simulink model "SOCPIControlBenchmarkRealDTOptimRand"  (R2019b)
settings: Solver=VariableStepAuto  StartTime=0.0  StopTime=tsim  FixedStep=0.01  RelTol=1e-3
values from neighbouring files (symbols this model uses):
  kio = 0.05    [benchmarkPIDStartRealOptimRand.m]
  kpo = 0.06    [benchmarkPIDStartRealOptimRand.m]
  maxKi = 0.1    [benchmarkPIDStartRealOptimRand.m]
  maxKp = 0.1    [benchmarkPIDStartRealOptimRand.m]
  minKi = 0.001    [benchmarkPIDStartRealOptimRand.m]
  minKp = 0.01    [benchmarkPIDStartRealOptimRand.m]
  optimPeriod = 300    [benchmarkPIDStartRealOptimRand.m]
  OVLim = 2    [benchmarkPIDStartRealOptimRand.m]
  refAmplitude = 50    [benchmarkPIDStartRealOptimRand.m]
  refSignalPeriod = 300    [benchmarkPIDStartRealOptimRand.m]
  resetThreshold = 0.1    [benchmarkPIDStartRealOptimRand.m]
  TSLim = 70    [benchmarkPIDStartRealOptimRand.m]
undefined symbols (not defined in the file or in its folder): conductance, FORandGCNM, resistance
libraries: fl_lib x28, nesl_utility x16, ee_lib x10, commchan3 x2, simulink x2, dspmathops x1
(part 1 of 2)
settings Model: SimulationMode=accelerator  Creator=jairo  LastModifiedBy=jairo
settings DataIOCC: ReturnWorkspaceOutputs=off

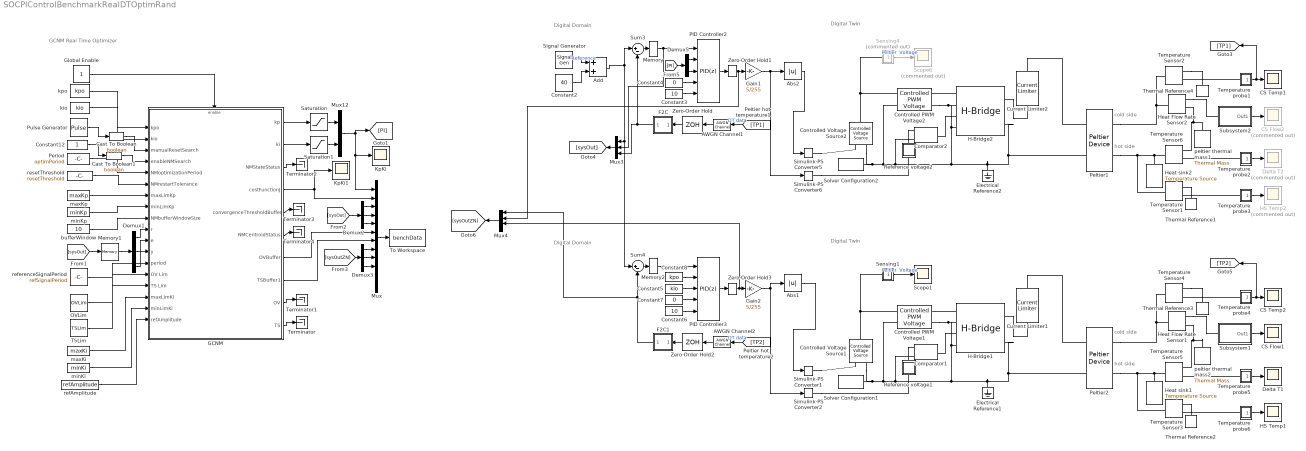
== system SOCPIControlBenchmarkRealDTOptimRand ==
  note: Digital Domain
  note: GCNM Real Time Optimizer
  note: hot side
  note: cold side
  note: Digital Twin
  note: Digital Twin
  note: hot side
  note: Digital Domain
  note: cold side
  AWGN Channel1 : commchan3/AWGN Channel  InputProcessing=Columns as channels (frame based)  seed=20  noiseMode=Variance from mask  EbNodB=10  EsNodB=10  SNRdB=10  bitsPerSym=1  Ps=1  Tsym=1  variance=0.01
      settings: SourceProductName=Communications Toolbox
  AWGN Channel2 : commchan3/AWGN Channel  InputProcessing=Columns as channels (frame based)  seed=20  noiseMode=Variance from mask  EbNodB=10  EsNodB=10  SNRdB=10  bitsPerSym=1  Ps=1  Tsym=1  variance=0.01
      settings: SourceProductName=Communications Toolbox
  Abs1 : Abs
  Abs2 : Abs
  Add : Sum
  CS Flow1 : Scope
  CS Flow2 : Scope  Commented=on
  CS Temp1 : Scope
  CS Temp2 : Scope
  Cast To Boolean : DataTypeConversion  OutDataTypeStr=boolean
  Cast To Boolean1 : DataTypeConversion  OutDataTypeStr=boolean
  Comparator1 : ee_lib/Integrated Circuits/Comparator  V_OS=5 mV  V_OL=0 V  V_OH=5 V  C_IN=0 pF  R_OUT=50 Ohm  Delay=0 s
      settings: SourceProductName=Simscape Electrical  SourceProductBaseCode=PS  InternalSimscapePortConfiguration="{\"Bottom\":[],\"Left\":[{\"id\":\"p\",\"label\":\"+\",\"type\":\"foundation.electrical.electrical\"},{\"id\":\"n\",\"label\":\"-\",\"type\":\"foundation.electrical.electrical\"}],\"Right\":[{\"id\":\"J\",\"label\":\"\",\"type\":\"foundation.electrical.electrical\"}],\"Top\":[]}"
  Comparator2 : ee_lib/Integrated Circuits/Comparator  V_OS=5 mV  V_OL=0 V  V_OH=5 V  C_IN=0 pF  R_OUT=50 Ohm  Delay=0 s
      settings: SourceProductName=Simscape Electrical  SourceProductBaseCode=PS  InternalSimscapePortConfiguration="{\"Bottom\":[],\"Left\":[{\"id\":\"p\",\"label\":\"+\",\"type\":\"foundation.electrical.electrical\"},{\"id\":\"n\",\"label\":\"-\",\"type\":\"foundation.electrical.electrical\"}],\"Right\":[{\"id\":\"J\",\"label\":\"\",\"type\":\"foundation.electrical.electrical\"}],\"Top\":[]}"
  Constant12 : Constant  OutDataTypeStr=boolean
  Constant2 : Constant  Value=40
  Constant3 : Constant  Value=10
  Constant4 : Constant  Value=0
  Constant5 : Constant  Value=kio
  Constant6 : Constant  Value=10
  Constant7 : Constant  Value=0
  Constant8 : Constant  Value=kpo
  Controlled PWM Voltage1 : ee_lib/Integrated Circuits/Controlled PWM Voltage  F=4000 Hz  TD=0 s  pulse_width_offset=0 s  pulse_min=0 s  Vmin=0 V  Vmax=5 V  Vm=5 V  pwm_or_av=2  event_type=1  sample_time=5e-6 s  u_min=0  u_max=1
      settings: SourceProductName=Simscape Electrical
  Controlled PWM Voltage2 : ee_lib/Integrated Circuits/Controlled PWM Voltage  F=4000 Hz  TD=0 s  pulse_width_offset=0 s  pulse_min=0 s  Vmin=0 V  Vmax=5 V  Vm=5 V  pwm_or_av=2  event_type=1  sample_time=5e-6 s  u_min=0  u_max=1
      settings: SourceProductName=Simscape Electrical
  Controlled Voltage Source1 : fl_lib/Electrical/Electrical Sources/Controlled Voltage Source
  Controlled Voltage Source2 : fl_lib/Electrical/Electrical Sources/Controlled Voltage Source
  Current Limiter1 : ee_lib/Semiconductors & Converters/Current Limiter  iLim=5 A  vLim=0.1 V  gLim=1e-3 1/Ohm  thermal_mass=100 J/K  initial_temperature=298.15 K
      settings: SourceProductName=Simscape Electrical  SourceProductBaseCode=PS  InternalSimscapePortConfiguration="{\"Bottom\":[],\"Left\":[{\"id\":\"p\",\"label\":\"+\",\"type\":\"foundation.electrical.electrical\"}],\"Right\":[{\"id\":\"n\",\"label\":\"-\",\"type\":\"foundation.electrical.electrical\"}],\"Top\":[]}"
  Current Limiter2 : ee_lib/Semiconductors & Converters/Current Limiter  iLim=5 A  vLim=0.1 V  gLim=1e-3 1/Ohm  thermal_mass=100 J/K  initial_temperature=298.15 K
      settings: SourceProductName=Simscape Electrical  SourceProductBaseCode=PS  InternalSimscapePortConfiguration="{\"Bottom\":[],\"Left\":[{\"id\":\"p\",\"label\":\"+\",\"type\":\"foundation.electrical.electrical\"}],\"Right\":[{\"id\":\"n\",\"label\":\"-\",\"type\":\"foundation.electrical.electrical\"}],\"Top\":[]}"
  Delta T1 : Scope
  Delta T2 : Scope  Commented=on
  Demux1 : Demux  Outputs=3
  Demux2 : Demux  Outputs=3
  Demux3 : Demux  Outputs=3
  Demux5 : Demux  Outputs=2
  Electrical Reference1 : fl_lib/Electrical/Electrical Elements/Electrical Reference
  Electrical Reference2 : fl_lib/Electrical/Electrical Elements/Electrical Reference
  F2C : Subsystem
  F2C1 : Subsystem
  GCNM : Subsystem
  Gain1 : Gain  Gain=5/255
  Gain2 : Gain  Gain=5/255
  Global Enable : Constant
  H-Bridge1 : ee_lib/Semiconductors & Converters/Converters/H-Bridge  supply_ports=ee.enum.supply_ports.hidesupply  Venable=2.5 V  Vmax=5 V  Vreverse=0.1 V  Vbrake=2.5 V  Vm=12 V  pwm_or_av=ee.enum.pwm_or_av.averaged  regenerative_braking_mode=ee.enum.converters.regenerative_braking_mode.always_enabled  discontinuous=ee.enum.current_profile.continuous  freewheeling_mode=ee.enum.converters.freewheeling_mode.one_switch_one_diode  Ron=0.1 Ohm  Don=0.1 Ohm  Goff=1e-6 S  Rload=3.38+0.1 Ohm  Lload=1e-5 H  F=4 kHz  thermal_mass=100 J/K  initial_temperature=298.15 K  Ron2=0.1 Ohm  Don2=0.05 Ohm  Tmeas=298.15 K  Tmeas2=398.15 K
      settings: SourceProductName=Simscape Electrical
  H-Bridge2 : ee_lib/Semiconductors & Converters/Converters/H-Bridge  supply_ports=ee.enum.supply_ports.hidesupply  Venable=2.5 V  Vmax=5 V  Vreverse=0.1 V  Vbrake=2.5 V  Vm=12 V  pwm_or_av=ee.enum.pwm_or_av.averaged  regenerative_braking_mode=ee.enum.converters.regenerative_braking_mode.always_enabled  discontinuous=ee.enum.current_profile.continuous  freewheeling_mode=ee.enum.converters.freewheeling_mode.one_switch_one_diode  Ron=0.1 Ohm  Don=0.1 Ohm  Goff=1e-6 S  Rload=3.38+0.1 Ohm  Lload=1e-5 H  F=4 kHz  thermal_mass=100 J/K  initial_temperature=298.15 K  Ron2=0.1 Ohm  Don2=0.05 Ohm  Tmeas=298.15 K  Tmeas2=398.15 K
      settings: SourceProductName=Simscape Electrical
  HS Temp1 : Scope
  HS Temp2 : Scope  Commented=on
  Heat Flow Rate Sensor1 : fl_lib/Thermal/Thermal Sensors/Heat Flow Rate Sensor
      settings: SourceProductName=Simscape  SourceProductBaseCode=SS
  Heat Flow Rate Sensor2 : fl_lib/Thermal/Thermal Sensors/Heat Flow Rate Sensor
      settings: SourceProductName=Simscape  SourceProductBaseCode=SS
  Heat sink1 : fl_lib/Thermal/Thermal Sources/Temperature Source  temperature=296 K
      settings: SourceProductName=Simscape
  Heat sink2 : fl_lib/Thermal/Thermal Sources/Temperature Source  temperature=296 K
      settings: SourceProductName=Simscape
  KpKi : Scope
  KpKi1 : Scope
  Memory : Memory
  Memory1 : Memory
  Memory2 : Memory
  Mux : Mux  Inputs=12
  Mux12 : Mux  Inputs=2
  Mux3 : Mux  Inputs=3
  Mux4 : Mux
  OVLim : Constant  Value=OVLim
  PID Controller2 : simulink/Continuous/PID Controller  Controller=PID  Form=Parallel  TimeDomain=Discrete-time  SampleTime=0.01  IntegratorMethod=Forward Euler  FilterMethod=Forward Euler  ControllerParametersSource=external  P=38.57  I=1.46877  D=6.66875  UseFilter=on  N=100  TunerSelectOption=Transfer Function Based (PID Tuner App)  InitialConditionSource=internal  InitialConditionForIntegrator=0  InitialConditionForFilter=0  DifferentiatorICPrevScaledInput=0  ExternalReset=none  TrackingMode=off  Kt=1  LimitOutput=on  UpperSaturationLimit=255  LowerSaturationLimit=-255  LinearizeAsGain=on  AntiWindupMode=back-calculation  Kb=1  POutMin=[]  POutMax=[]  IOutMin=[]  IOutMax=[]  DOutMin=[]  DOutMax=[]  NOutMin=[]  NOutMax=[]  SumOutMin=[]  SumOutMax=[]  SaturationOutMin=[]  SaturationOutMax=[]  PParamMin=[]  PParamMax=[]  IParamMin=[]  IParamMax=[]  DParamMin=[]  DParamMax=[]  NParamMin=[]  NParamMax=[]  KbParamMin=[]  KbParamMax=[]  KtParamMin=[]  KtParamMax=[]  KbOutMin=[]  KbOutMax=[]  KtOutMin=[]  KtOutMax=[]  IntegratorOutMin=[]  IntegratorOutMax=[]  FilterOutMin=[]  FilterOutMax=[]  SumI1OutMin=[]  SumI1OutMax=[]  SumI2OutMin=[]  SumI2OutMax=[]  SumI3OutMin=[]  SumI3OutMax=[]  SumI4OutMin=[]  SumI4OutMax=[]  SumDOutMin=[]  SumDOutMax=[]  DifferentiatorOutMin=[]  DifferentiatorOutMax=[]  FilterDiffOutCoefMin=[]  FilterDiffOutCoefMax=[]  ReciprocalOutMin=[]  ReciprocalOutMax=[]  SumDenOutMin=[]  SumDenOutMax=[]  SumNumOutMin=[]  SumNumOutMax=[]  DivideOutMin=[]  DivideOutMax=[]  IntegratorContinuousStateAttributes=''  IntegratorStateMustResolveToSignalObject=off  IntegratorRTWStateStorageClass=Auto  FilterContinuousStateAttributes=''  FilterStateMustResolveToSignalObject=off  FilterRTWStateStorageClass=Auto  ParallelPVariant=ExternalParameters  IdealPVariant=Disabled  IVariant=ExternalParameters  DVariant=ExternalParameters  IntegratorVariant=Discrete  SatVariant=Enabled  AWVariant=BackCalculation  PCopyVariant=Disabled  TRVariant=Disabled  FdbkBlocksVariant=Forward  IdealPFdbkVariant=Disabled  SatFdbkVariant=Disabled  DerivativeFilterVariant=ForwardEulerFilter  NVariant=ExternalParameters  NCopyVariant=Disabled  FilterICVariant=InternalICsFilter  IntegratorICVariant=InternalICs  ExternalResetVariant=Disabled  TRSumVariant=Passthrough  SumFdbkVariant=Disabled  SumVariant=Sum_PID
  PID Controller3 : simulink/Continuous/PID Controller  Controller=PID  Form=Parallel  TimeDomain=Discrete-time  SampleTime=0.01  IntegratorMethod=Forward Euler  FilterMethod=Forward Euler  ControllerParametersSource=external  P=38.57  I=1.46877  D=6.66875  UseFilter=on  N=100  TunerSelectOption=Transfer Function Based (PID Tuner App)  InitialConditionSource=internal  InitialConditionForIntegrator=0  InitialConditionForFilter=0  DifferentiatorICPrevScaledInput=0  ExternalReset=none  TrackingMode=off  Kt=1  LimitOutput=on  UpperSaturationLimit=255  LowerSaturationLimit=-255  LinearizeAsGain=on  AntiWindupMode=back-calculation  Kb=1  POutMin=[]  POutMax=[]  IOutMin=[]  IOutMax=[]  DOutMin=[]  DOutMax=[]  NOutMin=[]  NOutMax=[]  SumOutMin=[]  SumOutMax=[]  SaturationOutMin=[]  SaturationOutMax=[]  PParamMin=[]  PParamMax=[]  IParamMin=[]  IParamMax=[]  DParamMin=[]  DParamMax=[]  NParamMin=[]  NParamMax=[]  KbParamMin=[]  KbParamMax=[]  KtParamMin=[]  KtParamMax=[]  KbOutMin=[]  KbOutMax=[]  KtOutMin=[]  KtOutMax=[]  IntegratorOutMin=[]  IntegratorOutMax=[]  FilterOutMin=[]  FilterOutMax=[]  SumI1OutMin=[]  SumI1OutMax=[]  SumI2OutMin=[]  SumI2OutMax=[]  SumI3OutMin=[]  SumI3OutMax=[]  SumI4OutMin=[]  SumI4OutMax=[]  SumDOutMin=[]  SumDOutMax=[]  DifferentiatorOutMin=[]  DifferentiatorOutMax=[]  FilterDiffOutCoefMin=[]  FilterDiffOutCoefMax=[]  ReciprocalOutMin=[]  ReciprocalOutMax=[]  SumDenOutMin=[]  SumDenOutMax=[]  SumNumOutMin=[]  SumNumOutMax=[]  DivideOutMin=[]  DivideOutMax=[]  IntegratorContinuousStateAttributes=''  IntegratorStateMustResolveToSignalObject=off  IntegratorRTWStateStorageClass=Auto  FilterContinuousStateAttributes=''  FilterStateMustResolveToSignalObject=off  FilterRTWStateStorageClass=Auto  ParallelPVariant=ExternalParameters  IdealPVariant=Disabled  IVariant=ExternalParameters  DVariant=ExternalParameters  IntegratorVariant=Discrete  SatVariant=Enabled  AWVariant=BackCalculation  PCopyVariant=Disabled  TRVariant=Disabled  FdbkBlocksVariant=Forward  IdealPFdbkVariant=Disabled  SatFdbkVariant=Disabled  DerivativeFilterVariant=ForwardEulerFilter  NVariant=ExternalParameters  NCopyVariant=Disabled  FilterICVariant=InternalICsFilter  IntegratorICVariant=InternalICs  ExternalResetVariant=Disabled  TRSumVariant=Passthrough  SumFdbkVariant=Disabled  SumVariant=Sum_PID
  Peltier1 : ee_lib/Sensors & Transducers/Peltier Device  alpha=seebeck V/K  R=resistance Ohm  K=conductance W/K
      settings: SourceProductName=Simscape Electrical  SourceProductBaseCode=PS  InternalSimscapePortConfiguration="{\"Bottom\":[],\"Left\":[{\"id\":\"p\",\"label\":\"+\",\"type\":\"foundation.electrical.electrical\"},{\"id\":\"n\",\"label\":\"-\",\"type\":\"foundation.electrical.electrical\"}],\"Right\":[{\"id\":\"A\",\"label\":\"A\",\"type\":\"foundation.thermal.thermal\"},{\"id\":\"B\",\"label\":\"B\",\"type\":\"foundation.thermal.thermal\"}],\"Top\":[]}"
  Peltier2 : ee_lib/Sensors & Transducers/Peltier Device  alpha=seebeck V/K  R=resistance Ohm  K=conductance W/K
      settings: SourceProductName=Simscape Electrical  SourceProductBaseCode=PS  InternalSimscapePortConfiguration="{\"Bottom\":[],\"Left\":[{\"id\":\"p\",\"label\":\"+\",\"type\":\"foundation.electrical.electrical\"},{\"id\":\"n\",\"label\":\"-\",\"type\":\"foundation.electrical.electrical\"}],\"Right\":[{\"id\":\"A\",\"label\":\"A\",\"type\":\"foundation.thermal.thermal\"},{\"id\":\"B\",\"label\":\"B\",\"type\":\"foundation.thermal.thermal\"}],\"Top\":[]}"
  Period : Constant  Value=optimPeriod  OutDataTypeStr=double
  Pulse Generator : DiscretePulseGenerator  PulseType=Time based  Period=20  PulseWidth=0.1
  Reference voltage1 : Subsystem
      mask Display: disp('Vr')
  Reference voltage2 : Subsystem
      mask Display: disp('Vr')
  Saturation : Saturate  UpperLimit=200  LowerLimit=0
  Saturation1 : Saturate  UpperLimit=200  LowerLimit=0
  Scope1 : Scope
  Scope6 : Scope  Commented=on
  Sensing1 : Subsystem
      mask Display: disp('V')
  Sensing4 : Subsystem  Commented=on
      mask Display: disp('V')
  Signal Generator : SignalGenerator  WaveForm=square  Amplitude=10  Frequency=1/refSignalPeriod
  Simulink-PS Converter{1..2,5..6} (4 alike) : nesl_utility/Simulink-PS Converter  PhysicalDomain=network_engine_domain  SubClassName=ps_input  LeftPortType=input  RightPortType=output  PseudoPeriodic=off  Frequencies=[]  NoiseDistribution=none  NoiseParameters=[]  Unit=1  AffineConversion=off  FilteringAndDerivatives=provide  SimscapeFilterOrder=1  InputFilterTimeConstant=0.001  UdotUserProvided=0
  Solver Configuration1 : nesl_utility/Solver Configuration  PhysicalDomain=network_engine_domain  SubClassName=solver  LeftPortType=input  RightPortType=generic  Tones=[]  Harmonics=[]  SimulateNoise=off  Profile=off  UseLocalSampling=off  EnableSwitchedLinearOptims=on  FrequencyDomain=off  UseCCode=off  RelTol=0.001  AbsTol=1e-06  MinStep=1e-09  ToWorkspace=off  RevertToSquareIcSolve=off  NumHomotopyIterations=100  PhasorMode=off  PhasorModeNumHarmonics=1  DoDC=off  ResidualTolerance=1e-09  UseLocalSolver=off  LocalSolverChoice=NE_BACKWARD_EULER_ADVANCER  LocalSolverSampleTime=0.001  DoFixedCost=off  MaxNonlinIter=3  MaxModeIter=2  LinearAlgebra=auto  EquationFormulation=NE_TIME_EF  DelaysMemoryBudget=1024  AutomaticFiltering=on  FilteringTimeConstant=0.01  PartitionStorageMethod=AS_NEEDED  PartitionMemoryBudget=1024  PartitionMethod=FAST
  Solver Configuration2 : nesl_utility/Solver Configuration  PhysicalDomain=network_engine_domain  SubClassName=solver  LeftPortType=input  RightPortType=generic  Tones=[]  Harmonics=[]  SimulateNoise=off  Profile=off  UseLocalSampling=off  EnableSwitchedLinearOptims=on  FrequencyDomain=off  UseCCode=off  RelTol=0.001  AbsTol=1e-06  MinStep=1e-09  ToWorkspace=off  RevertToSquareIcSolve=off  NumHomotopyIterations=100  PhasorMode=off  PhasorModeNumHarmonics=1  DoDC=off  ResidualTolerance=1e-09  UseLocalSolver=off  LocalSolverChoice=NE_BACKWARD_EULER_ADVANCER  LocalSolverSampleTime=0.001  DoFixedCost=off  MaxNonlinIter=3  MaxModeIter=2  LinearAlgebra=auto  EquationFormulation=NE_TIME_EF  DelaysMemoryBudget=1024  AutomaticFiltering=on  FilteringTimeConstant=0.01  PartitionStorageMethod=AS_NEEDED  PartitionMemoryBudget=1024  PartitionMethod=FAST
  Subsystem1 : Subsystem
      mask Display: disp('Heat flow')
  Subsystem2 : Subsystem
      mask Display: disp('Heat flow')
  Sum3 : Sum  Inputs=|+-
  Sum4 : Sum  Inputs=|+-
  TSLim : Constant  Value=TSLim
  Temperature Sensor{1..6} (6 alike) : fl_lib/Thermal/Thermal Sensors/Temperature Sensor
  Temperature probe1 : Subsystem
      mask Display: disp('T')
  Temperature probe2 : Subsystem
      mask Display: disp('T')
  Temperature probe3 : Subsystem
      mask Display: disp('T')
  Temperature probe4 : Subsystem
      mask Display: disp('T')
  Temperature probe5 : Subsystem
      mask Display: disp('T')
  Temperature probe6 : Subsystem
      mask Display: disp('T')
  Terminator{,1..4} (5 alike) : Terminator
  Thermal Reference{1..4} (4 alike) : fl_lib/Thermal/Thermal Elements/Thermal Reference
  To Workspace : ToWorkspace  VariableName=benchData  SaveFormat=Timeseries  SampleTime=-1
  Zero-Order Hold : ZeroOrderHold  SampleTime=-1
  Zero-Order Hold1 : ZeroOrderHold
  Zero-Order Hold2 : ZeroOrderHold  SampleTime=-1
  Zero-Order Hold3 : ZeroOrderHold
  bufferWindow : Constant  Value=10  OutDataTypeStr=uint16
  kio : Constant  Value=kio  OutDataTypeStr=double
  kpo : Constant  Value=kpo  OutDataTypeStr=double
  maxKi : Constant  Value=maxKi  VectorParams1D=off  OutDataTypeStr=double
  maxKp : Constant  Value=maxKp  OutDataTypeStr=double
  minKi : Constant  Value=minKi  OutDataTypeStr=double
  minKp : Constant  Value=minKp  OutDataTypeStr=double
  peltier thermal mass1 : fl_lib/Thermal/Thermal Elements/Thermal Mass  mass=1 kg  sp_heat=Cp J/kg/K  T_specify=on  T_priority=High  T=296 K  T_nominal_specify=off  T_nominal_unit=K  T_nominal_value=1  Q_specify=off  Q_priority=Low  Q=0 W  Q_nominal_specify=off  Q_nominal_unit=W  Q_nominal_value=1
  peltier thermal mass2 : fl_lib/Thermal/Thermal Elements/Thermal Mass  mass=1 kg  sp_heat=Cp J/kg/K  T_specify=on  T_priority=High  T=296 K  T_nominal_specify=off  T_nominal_unit=K  T_nominal_value=1  Q_specify=off  Q_priority=Low  Q=0 W  Q_nominal_specify=off  Q_nominal_unit=W  Q_nominal_value=1
  refAmplitude : Constant  Value=refAmplitude  OutDataTypeStr=double
  referenceSignalPeriod : Constant  Value=refSignalPeriod
  resetThreshold : Constant  Value=resetThreshold
  wires:
  resetThreshold/1 -> GCNM/6(NMrestartTolerance)
  Mux12/1 -> [PI], Mux/1, KpKi/1
  maxKp/1 -> GCNM/7(maxLimKp)
  bufferWindow/1 -> GCNM/9(NMbufferWindowSize)
  Cast To Boolean1/1 -> GCNM/4(enableNMSearch)
  kio/1 -> GCNM/2(kio)
  Pulse Generator/1 -> Cast To Boolean/1
  Cast To Boolean/1 -> GCNM/3(manualResetSearch)
  Constant12/1 -> Cast To Boolean1/1
  minKp/1 -> GCNM/8(minLimKp)
  Global Enable/1 -> GCNM/Enable
  kpo/1 -> GCNM/1(kpo)
  Period/1 -> GCNM/5(NMoptimizationPeriod)
  GCNM/4(costFunctionJ) -> Mux/2, KpKi1/1
  referenceSignalPeriod/1 -> GCNM/13("  period")
  OVLim/1 -> GCNM/14("  OV Lim")
  TSLim/1 -> GCNM/15(TS Lim)
  GCNM/1("  kp") -> Saturation/1
  GCNM/2("  ki") -> Saturation1/1
  Mux/1 -> To Workspace/1
  maxKi/1 -> GCNM/16(maxLimKi)
  minKi/1 -> GCNM/17(minLimKi)
  [sysOut] -> Memory1/1
  Demux1/1 -> GCNM/10("  r")
  Demux1/2 -> GCNM/11("  e")
  Demux1/3 -> GCNM/12("  y")
  [sysOut] -> Demux2/1
  Demux2/1 -> Mux/3
  Demux2/2 -> Mux/4
  Demux2/3 -> Mux/5
  [sysOutZN] -> Demux3/1
  Demux3/1 -> Mux/8
  Demux3/2 -> Mux/9
  Demux3/3 -> Mux/10
  GCNM/10(TS) -> Terminator/1
  GCNM/9(OV) -> Terminator1/1
  GCNM/8(TSBuffer1) -> Mux/7
  GCNM/7(OVBuffer) -> Mux/6
  GCNM/3(NMStateStatus) -> Terminator2/1
  GCNM/5(convergenceThresholdBuffer) -> Terminator3/1
  GCNM/6(NMCentroidStatus) -> Terminator4/1
  Signal Generator/1 -> Add/1  "Reference"
  Constant2/1 -> Add/2
  refAmplitude/1 -> GCNM/18(refAmplitude)
  Sensing4/1(Out1) -> Scope6/1  "Peltier  Voltage"
  Zero-Order Hold1/1 -> Mux4/2, Gain1/1
  Temperature probe1/1(K) -> [TP1], CS Temp1/1
  [TP1] -> AWGN Channel1/1  "DT data"
  PID Controller2/1 -> Zero-Order Hold1/1
  Temperature probe2/1(K) -> Delta T2/1
  Subsystem2/1(Out1) -> CS Flow2/1
  Gain1/1 -> Abs2/1, Simulink-PS Converter6/1
  Abs2/1 -> Simulink-PS Converter5/1
  Temperature probe3/1(K) -> HS Temp2/1
  AWGN Channel1/1 -> Zero-Order Hold/1
  Mux3/1 -> [sysOut]
  Constant4/1 -> PID Controller2/4
  Constant3/1 -> PID Controller2/5
  Zero-Order Hold/1 -> F2C/1(In1)
  Sum3/1 -> Memory/1
  Memory/1 -> Mux3/2, PID Controller2/1
  [PI] -> Demux5/1
  Demux5/1 -> PID Controller2/2
  Demux5/2 -> PID Controller2/3
  Memory1/1 -> Demux1/1
  F2C/1(Out1) -> Mux3/3, Sum3/2
  Temperature probe5/1(K) -> Delta T1/1
  PID Controller3/1 -> Zero-Order Hold3/1
  Zero-Order Hold3/1 -> Mux4/3, Gain2/1
  Temperature probe4/1(K) -> [TP2], CS Temp2/1
  Sensing1/1(Out1) -> Scope1/1  "Peltier  Voltage"
  Sum4/1 -> Memory2/1
  Abs1/1 -> Simulink-PS Converter1/1
  AWGN Channel2/1 -> Zero-Order Hold2/1
  Add/1 -> Sum4/1, Mux3/1, Sum3/1
  Gain2/1 -> Abs1/1, Simulink-PS Converter2/1
  Zero-Order Hold2/1 -> F2C1/1(In1)
  Subsystem1/1(Out1) -> CS Flow1/1
  [TP2] -> AWGN Channel2/1  "DT data"
  F2C1/1(Out1) -> Mux4/1, Sum4/2
  Constant7/1 -> PID Controller3/4
  Memory2/1 -> PID Controller3/1
  Temperature probe6/1(K) -> HS Temp1/1
  Constant6/1 -> PID Controller3/5
  Mux4/1 -> [sysOutZN]
  Constant8/1 -> PID Controller3/2
  Constant5/1 -> PID Controller3/3
  Saturation/1 -> Mux12/1
  Saturation1/1 -> Mux12/2
  connections:
  Controlled PWM Voltage2/LConn1 -- Controlled Voltage Source2/LConn1 -- Sensing4/LConn1
  Peltier1/RConn1 -- Heat Flow Rate Sensor2/LConn1 -- Temperature Sensor2/LConn1
  Controlled PWM Voltage2/RConn2 -- Peltier1/LConn2 -- H-Bridge2/RConn2 -- Electrical Reference2/LConn1 -- Comparator2/LConn2 -- Controlled Voltage Source2/RConn2 -- Solver Configuration2/RConn1 -- Controlled PWM Voltage2/LConn2 -- H-Bridge2/LConn4 -- H-Bridge2/LConn2
  peltier thermal mass1/LConn1 -- Temperature Sensor6/RConn1 -- Heat Flow Rate Sensor2/RConn2
  Heat sink2/LConn1 -- Temperature Sensor6/LConn1 -- Peltier1/RConn2 -- Temperature Sensor1/LConn1
  Peltier1/LConn1 -- Current Limiter2/RConn1
  Simulink-PS Converter6/RConn1 -- Reference voltage2/RConn1
  Temperature Sensor2/RConn1 -- Thermal Reference4/LConn1
  Temperature Sensor1/RConn1 -- Thermal Reference1/LConn1
  Heat Flow Rate Sensor2/RConn1 -- Subsystem2/LConn1
  Comparator2/RConn1 -- H-Bridge2/LConn3
  Reference voltage2/LConn1 -- Comparator2/LConn1
  Temperature probe1/LConn1 -- Temperature Sensor2/RConn2
  Temperature probe3/LConn1 -- Temperature Sensor1/RConn2
  Temperature probe2/LConn1 -- Temperature Sensor6/RConn2
  H-Bridge2/RConn1 -- Current Limiter2/LConn1
  Simulink-PS Converter5/RConn1 -- Controlled Voltage Source2/RConn1
  H-Bridge2/LConn1 -- Controlled PWM Voltage2/RConn1
  Controlled PWM Voltage1/RConn2 -- H-Bridge1/LConn2 -- H-Bridge1/LConn4 -- Peltier2/LConn2 -- H-Bridge1/RConn2 -- Electrical Reference1/LConn1 -- Comparator1/LConn2 -- Controlled Voltage Source1/RConn2 -- Solver Configuration1/RConn1 -- Controlled PWM Voltage1/LConn2
  Heat sink1/LConn1 -- Temperature Sensor5/LConn1 -- Peltier2/RConn2 -- Temperature Sensor3/LConn1
  Peltier2/RConn1 -- Heat Flow Rate Sensor1/LConn1 -- Temperature Sensor4/LConn1
  peltier thermal mass2/LConn1 -- Temperature Sensor5/RConn1 -- Heat Flow Rate Sensor1/RConn2
  Controlled PWM Voltage1/LConn1 -- Controlled Voltage Source1/LConn1 -- Sensing1/LConn1
  Peltier2/LConn1 -- Current Limiter1/RConn1
  Temperature probe4/LConn1 -- Temperature Sensor4/RConn2
  Heat Flow Rate Sensor1/RConn1 -- Subsystem1/LConn1
  Temperature Sensor3/RConn1 -- Thermal Reference2/LConn1
  Temperature Sensor4/RConn1 -- Thermal Reference3/LConn1
  Reference voltage1/LConn1 -- Comparator1/LConn1
  Simulink-PS Converter2/RConn1 -- Reference voltage1/RConn1
  H-Bridge1/LConn1 -- Controlled PWM Voltage1/RConn1
  Temperature probe5/LConn1 -- Temperature Sensor5/RConn2
  Comparator1/RConn1 -- H-Bridge1/LConn3
  H-Bridge1/RConn1 -- Current Limiter1/LConn1
  Temperature probe6/LConn1 -- Temperature Sensor3/RConn2
  Simulink-PS Converter1/RConn1 -- Controlled Voltage Source1/RConn1

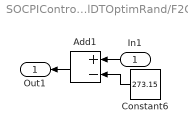
== system SOCPIControlBenchmarkRealDTOptimRand/F2C ==
  In1 : Inport
  Add1 : Sum  Inputs=+-
  Constant6 : Constant  Value=273.15
  Out1 : Outport
  wires:
  Add1/1 -> Out1/1
  Constant6/1 -> Add1/2
  In1/1 -> Add1/1

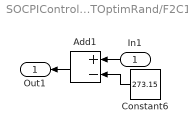
== system SOCPIControlBenchmarkRealDTOptimRand/F2C1 ==
  In1 : Inport
  Add1 : Sum  Inputs=+-
  Constant6 : Constant  Value=273.15
  Out1 : Outport
  wires:
  Add1/1 -> Out1/1
  Constant6/1 -> Add1/2
  In1/1 -> Add1/1

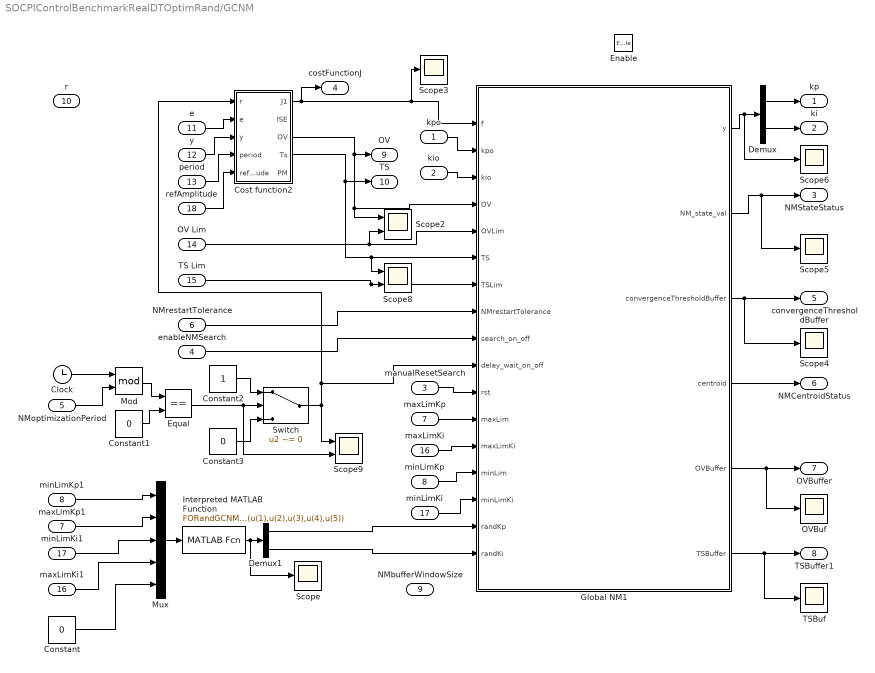
== system SOCPIControlBenchmarkRealDTOptimRand/GCNM ==
  kpo : Inport  OutDataTypeStr=double
  kio : Inport  Port=2  OutDataTypeStr=double
  manualResetSearch : Inport  Port=3  OutDataTypeStr=boolean
  enableNMSearch : Inport  Port=4  OutDataTypeStr=boolean
  NMoptimizationPeriod : Inport  Port=5  OutDataTypeStr=double
  NMrestartTolerance : Inport  Port=6
  maxLimKp : Inport  Port=7  OutDataTypeStr=double
  minLimKp : Inport  Port=8  OutDataTypeStr=double
  NMbufferWindowSize : Inport  Port=9  OutDataTypeStr=uint16
  "  r" : Inport  Port=10  OutDataTypeStr=double
  "  e" : Inport  Port=11  OutDataTypeStr=double
  "  y" : Inport  Port=12  OutDataTypeStr=double
  "  period" : Inport  Port=13  OutDataTypeStr=double
  "  OV Lim" : Inport  Port=14  OutDataTypeStr=double
  TS Lim : Inport  Port=15  OutDataTypeStr=double
  maxLimKi : Inport  Port=16  OutDataTypeStr=double
  minLimKi : Inport  Port=17  OutDataTypeStr=double
  refAmplitude : Inport  Port=18  OutDataTypeStr=double
  Enable : EnablePort
  Clock : Clock
  Constant : Constant  Value=0
  Constant1 : Constant  Value=0
  Constant2 : Constant
  Constant3 : Constant  Value=0
  Cost function2 : Subsystem
  Demux : Demux  Outputs=2
  Demux1 : Demux  Outputs=2
  Equal : RelationalOperator  Operator===  RndMeth=Simplest
  Global NM1 : MATLAB Function  TreatAsAtomicUnit=on
  Interpreted MATLAB Function : MATLABFcn  MATLABFcn=FORandGCNM(u(1),u(2),u(3),u(4),u(5))  OutputDimensions=2
  Mod : Math  Operator=mod  SignedPower=off  SaturateOnIntegerOverflow=on
  Mux : Mux  Inputs=5
  OVBuf : Scope
  Scope{,3..6} (5 alike) : Scope
  Scope2 : Scope  NumInputPorts=2
  Scope8 : Scope  NumInputPorts=2
  Scope9 : Scope  NumInputPorts=2
  Switch : Switch  Criteria=u2 ~= 0
  TSBuf : Scope
  maxLimKi1 : InportShadow  Port=16  OutDataTypeStr=double
  maxLimKp1 : InportShadow  Port=7  OutDataTypeStr=double
  minLimKi1 : InportShadow  Port=17  OutDataTypeStr=double
  minLimKp1 : InportShadow  Port=8  OutDataTypeStr=double
  "  kp" : Outport  OutDataTypeStr=double
  "  ki" : Outport  Port=2  OutDataTypeStr=double
  NMStateStatus : Outport  Port=3  OutDataTypeStr=double
  costFunctionJ : Outport  Port=4  OutDataTypeStr=double
  convergenceThresholdBuffer : Outport  Port=5  OutDataTypeStr=double
  NMCentroidStatus : Outport  Port=6  OutDataTypeStr=double
  OVBuffer : Outport  Port=7  OutDataTypeStr=double
  TSBuffer1 : Outport  Port=8  OutDataTypeStr=double
  OV : Outport  Port=9  OutDataTypeStr=double
  TS : Outport  Port=10  OutDataTypeStr=double
  wires:
  Demux/2 -> "  ki"/1
  Demux/1 -> "  kp"/1
  NMrestartTolerance/1 -> Global NM1/8(NMrestartTolerance)
  manualResetSearch/1 -> Global NM1/11(rst)
  enableNMSearch/1 -> Global NM1/9(search_on_off)
  minLimKp/1 -> Global NM1/14(minLim)
  maxLimKp/1 -> Global NM1/12(maxLim)
  Global NM1/2(NM_state_val) -> Scope5/1, NMStateStatus/1
  Global NM1/3(convergenceThresholdBuffer) -> Scope4/1, convergenceThresholdBuffer/1
  Global NM1/4(centroid) -> NMCentroidStatus/1
  Global NM1/1(y) -> Scope6/1, Demux/1
  kpo/1 -> Global NM1/2(kpo)
  kio/1 -> Global NM1/3(kio)
  Cost function2/3(OV) -> OV/1, Global NM1/4(OV), Scope2/1
  "  y"/1 -> Cost function2/3(y)
  "  e"/1 -> Cost function2/2(e)
  Global NM1/5(OVBuffer) -> OVBuf/1, OVBuffer/1
  "  period"/1 -> Cost function2/4(period)
  "  OV Lim"/1 -> Scope2/2, Global NM1/5(OVLim)
  Cost function2/4(Ts) -> TS/1, Global NM1/6(TS), Scope8/1
  TS Lim/1 -> Global NM1/7(TSLim), Scope8/2
  Global NM1/6(TSBuffer) -> TSBuf/1, TSBuffer1/1
  Cost function2/1(J1) -> Scope3/1, Global NM1/1(f), costFunctionJ/1
  Clock/1 -> Mod/1
  NMoptimizationPeriod/1 -> Mod/2
  Constant1/1 -> Equal/2
  Mod/1 -> Equal/1
  Constant2/1 -> Switch/1
  Constant3/1 -> Switch/3
  Switch/1 -> Scope9/1, Cost function2/1(r), Global NM1/10(delay_wait_on_off)
  Equal/1 -> Scope9/2, Switch/2
  maxLimKi/1 -> Global NM1/13(maxLimKi)
  minLimKi/1 -> Global NM1/15(minLimKi)
  refAmplitude/1 -> Cost function2/5(refAmplitude)
  Mux/1 -> Interpreted MATLAB Function/1
  minLimKp1/1 -> Mux/1
  maxLimKp1/1 -> Mux/2
  Interpreted MATLAB Function/1 -> Scope/1, Demux1/1
  Demux1/1 -> Global NM1/16(randKp)
  Demux1/2 -> Global NM1/17(randKi)
  Constant/1 -> Mux/5
  maxLimKi1/1 -> Mux/4
  minLimKi1/1 -> Mux/3

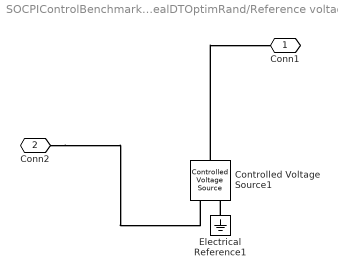
== system SOCPIControlBenchmarkRealDTOptimRand/Reference voltage1 ==
  Controlled Voltage Source1 : fl_lib/Electrical/Electrical Sources/Controlled Voltage Source
  Electrical Reference1 : fl_lib/Electrical/Electrical Elements/Electrical Reference
  Conn1 : PMIOPort  Side=Left
  Conn2 : PMIOPort  Port=2  Side=Right
  connections:
  Electrical Reference1/LConn1 -- Controlled Voltage Source1/RConn2
  Controlled Voltage Source1/LConn1 -- Conn1/RConn1
  Conn2/RConn1 -- Controlled Voltage Source1/RConn1

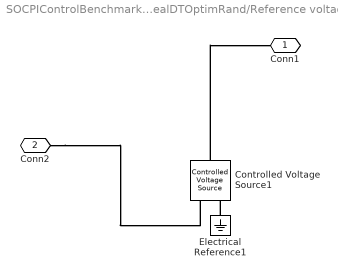
== system SOCPIControlBenchmarkRealDTOptimRand/Reference voltage2 ==
  Controlled Voltage Source1 : fl_lib/Electrical/Electrical Sources/Controlled Voltage Source
  Electrical Reference1 : fl_lib/Electrical/Electrical Elements/Electrical Reference
  Conn1 : PMIOPort  Side=Left
  Conn2 : PMIOPort  Port=2  Side=Right
  connections:
  Electrical Reference1/LConn1 -- Controlled Voltage Source1/RConn2
  Controlled Voltage Source1/LConn1 -- Conn1/RConn1
  Conn2/RConn1 -- Controlled Voltage Source1/RConn1

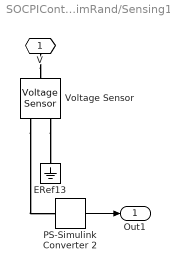
== system SOCPIControlBenchmarkRealDTOptimRand/Sensing1 ==
  ERef13 : fl_lib/Electrical/Electrical Elements/Electrical Reference
  PS-Simulink Converter 2 : nesl_utility/PS-Simulink Converter  PhysicalDomain=network_engine_domain  SubClassName=ps_output  LeftPortType=input  RightPortType=output  PseudoPeriodic=off  Frequencies=[]  Unit=V  AffineConversion=off
  Voltage Sensor : fl_lib/Electrical/Electrical Sensors/Voltage Sensor
  V : PMIOPort  Side=Left
  Out1 : Outport  VectorParamsAs1DForOutWhenUnconnected=off
  wires:
  PS-Simulink Converter 2/1 -> Out1/1
  connections:
  V/RConn1 -- Voltage Sensor/LConn1
  Voltage Sensor/RConn2 -- ERef13/LConn1
  Voltage Sensor/RConn1 -- PS-Simulink Converter 2/LConn1

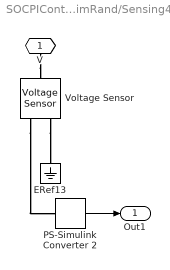
== system SOCPIControlBenchmarkRealDTOptimRand/Sensing4 ==
  ERef13 : fl_lib/Electrical/Electrical Elements/Electrical Reference
  PS-Simulink Converter 2 : nesl_utility/PS-Simulink Converter  PhysicalDomain=network_engine_domain  SubClassName=ps_output  LeftPortType=input  RightPortType=output  PseudoPeriodic=off  Frequencies=[]  Unit=V  AffineConversion=off
  Voltage Sensor : fl_lib/Electrical/Electrical Sensors/Voltage Sensor
  V : PMIOPort  Side=Left
  Out1 : Outport  VectorParamsAs1DForOutWhenUnconnected=off
  wires:
  PS-Simulink Converter 2/1 -> Out1/1
  connections:
  V/RConn1 -- Voltage Sensor/LConn1
  Voltage Sensor/RConn2 -- ERef13/LConn1
  Voltage Sensor/RConn1 -- PS-Simulink Converter 2/LConn1

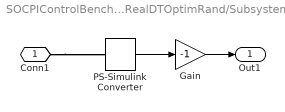
== system SOCPIControlBenchmarkRealDTOptimRand/Subsystem1 ==
  Gain : Gain  Gain=-1
  PS-Simulink Converter : nesl_utility/PS-Simulink Converter  PhysicalDomain=network_engine_domain  SubClassName=ps_output  LeftPortType=input  RightPortType=output  PseudoPeriodic=off  Frequencies=[]  Unit=J/s  AffineConversion=off
  Conn1 : PMIOPort  Side=Left
  Out1 : Outport  VectorParamsAs1DForOutWhenUnconnected=off
  wires:
  Gain/1 -> Out1/1
  PS-Simulink Converter/1 -> Gain/1
  connections:
  Conn1/RConn1 -- PS-Simulink Converter/LConn1

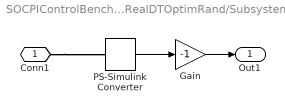
== system SOCPIControlBenchmarkRealDTOptimRand/Subsystem2 ==
  Gain : Gain  Gain=-1
  PS-Simulink Converter : nesl_utility/PS-Simulink Converter  PhysicalDomain=network_engine_domain  SubClassName=ps_output  LeftPortType=input  RightPortType=output  PseudoPeriodic=off  Frequencies=[]  Unit=J/s  AffineConversion=off
  Conn1 : PMIOPort  Side=Left
  Out1 : Outport  VectorParamsAs1DForOutWhenUnconnected=off
  wires:
  Gain/1 -> Out1/1
  PS-Simulink Converter/1 -> Gain/1
  connections:
  Conn1/RConn1 -- PS-Simulink Converter/LConn1

== system SOCPIControlBenchmarkRealDTOptimRand/Temperature probe1 ==
  Gain : Gain
  PS-Simulink Converter : nesl_utility/PS-Simulink Converter  PhysicalDomain=network_engine_domain  SubClassName=ps_output  LeftPortType=input  RightPortType=output  PseudoPeriodic=off  Frequencies=[]  Unit=K  AffineConversion=off
  ThermalFlow : PMIOPort  Side=Left
  K : Outport
  wires:
  PS-Simulink Converter/1 -> Gain/1
  Gain/1 -> K/1
  connections:
  PS-Simulink Converter/LConn1 -- ThermalFlow/RConn1

== system SOCPIControlBenchmarkRealDTOptimRand/Temperature probe2 ==
  Gain : Gain
  PS-Simulink Converter : nesl_utility/PS-Simulink Converter  PhysicalDomain=network_engine_domain  SubClassName=ps_output  LeftPortType=input  RightPortType=output  PseudoPeriodic=off  Frequencies=[]  Unit=K  AffineConversion=off
  ThermalFlow : PMIOPort  Side=Left
  K : Outport
  wires:
  PS-Simulink Converter/1 -> Gain/1
  Gain/1 -> K/1
  connections:
  PS-Simulink Converter/LConn1 -- ThermalFlow/RConn1

== system SOCPIControlBenchmarkRealDTOptimRand/Temperature probe3 ==
  Gain : Gain
  PS-Simulink Converter : nesl_utility/PS-Simulink Converter  PhysicalDomain=network_engine_domain  SubClassName=ps_output  LeftPortType=input  RightPortType=output  PseudoPeriodic=off  Frequencies=[]  Unit=K  AffineConversion=off
  ThermalFlow : PMIOPort  Side=Left
  K : Outport
  wires:
  PS-Simulink Converter/1 -> Gain/1
  Gain/1 -> K/1
  connections:
  PS-Simulink Converter/LConn1 -- ThermalFlow/RConn1

== system SOCPIControlBenchmarkRealDTOptimRand/Temperature probe4 ==
  Gain : Gain
  PS-Simulink Converter : nesl_utility/PS-Simulink Converter  PhysicalDomain=network_engine_domain  SubClassName=ps_output  LeftPortType=input  RightPortType=output  PseudoPeriodic=off  Frequencies=[]  Unit=K  AffineConversion=off
  ThermalFlow : PMIOPort  Side=Left
  K : Outport
  wires:
  PS-Simulink Converter/1 -> Gain/1
  Gain/1 -> K/1
  connections:
  PS-Simulink Converter/LConn1 -- ThermalFlow/RConn1

== system SOCPIControlBenchmarkRealDTOptimRand/Temperature probe5 ==
  Gain : Gain
  PS-Simulink Converter : nesl_utility/PS-Simulink Converter  PhysicalDomain=network_engine_domain  SubClassName=ps_output  LeftPortType=input  RightPortType=output  PseudoPeriodic=off  Frequencies=[]  Unit=K  AffineConversion=off
  ThermalFlow : PMIOPort  Side=Left
  K : Outport
  wires:
  PS-Simulink Converter/1 -> Gain/1
  Gain/1 -> K/1
  connections:
  PS-Simulink Converter/LConn1 -- ThermalFlow/RConn1

== system SOCPIControlBenchmarkRealDTOptimRand/Temperature probe6 ==
  Gain : Gain
  PS-Simulink Converter : nesl_utility/PS-Simulink Converter  PhysicalDomain=network_engine_domain  SubClassName=ps_output  LeftPortType=input  RightPortType=output  PseudoPeriodic=off  Frequencies=[]  Unit=K  AffineConversion=off
  ThermalFlow : PMIOPort  Side=Left
  K : Outport
  wires:
  PS-Simulink Converter/1 -> Gain/1
  Gain/1 -> K/1
  connections:
  PS-Simulink Converter/LConn1 -- ThermalFlow/RConn1

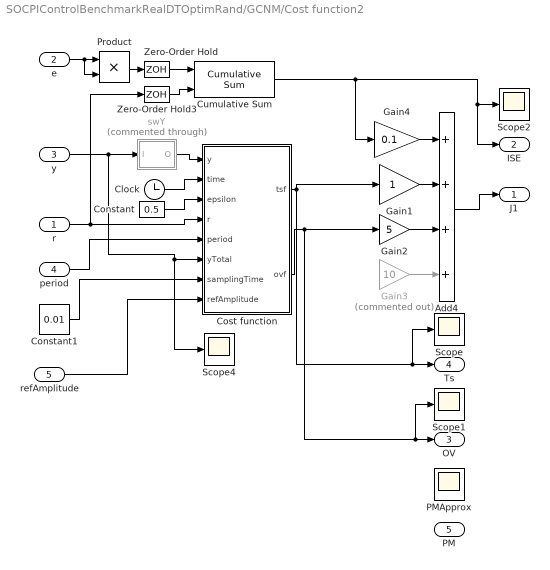
== system SOCPIControlBenchmarkRealDTOptimRand/GCNM/Cost function2 ==
  r : Inport
  e : Inport  Port=2
  y : Inport  Port=3
  period : Inport  Port=4
  refAmplitude : Inport  Port=5
  Add4 : Sum  Inputs=++++
  Clock : Clock
  Constant : Constant  Value=0.5
  Constant1 : Constant  Value=0.01
  Cost function : MATLAB Function  TreatAsAtomicUnit=on
  Cumulative Sum : dspmathops/Cumulative Sum  dim=Channels (running sum)  InputProcessing=Columns as channels (frame based)  reset_popup=Falling edge  roundingMode=Floor  overflowMode=off  outputDataTypeStr=Inherit: Same as accumulator  outputMin=[]  outputMax=[]  outputLastDataTypeStr=Inherit: Same as accumulator
      settings: SourceProductName=DSP System Toolbox
  Gain1 : Gain
  Gain2 : Gain  Gain=5
  Gain3 : Gain  Commented=on  Gain=10
  Gain4 : Gain  Gain=0.1
  PMApprox : Scope
  Product : Product
  Scope{,1..2,4} (4 alike) : Scope
  Zero-Order Hold : ZeroOrderHold  SampleTime=-1
  Zero-Order Hold3 : ZeroOrderHold  SampleTime=-1
  swY : Subsystem  Commented=through
  J1 : Outport
  ISE : Outport  Port=2
  OV : Outport  Port=3
  Ts : Outport  Port=4
  PM : Outport  Port=5
  wires:
  Cumulative Sum/1 -> Gain4/1, ISE/1, Scope2/1
  Zero-Order Hold3/1 -> Cumulative Sum/2
  e/1 -> Product/2, Product/1
  Zero-Order Hold/1 -> Cumulative Sum/1
  r/1 -> Zero-Order Hold3/1, Cost function/4(r)
  swY/1(O) -> Cost function/1(y)
  Clock/1 -> Cost function/2(time)
  Product/1 -> Zero-Order Hold/1
  Constant/1 -> Cost function/3(epsilon)
  y/1 -> Scope4/1, Cost function/6(yTotal), swY/1(I)
  Add4/1 -> J1/1
  Gain2/1 -> Add4/3
  period/1 -> Cost function/5(period)
  Constant1/1 -> Cost function/7(samplingTime)
  Gain1/1 -> Add4/2
  refAmplitude/1 -> Cost function/8(refAmplitude)
  Gain3/1 -> Add4/4
  Cost function/1(tsf) -> Gain1/1, Scope/1, Ts/1
  Cost function/2(ovf) -> Scope1/1, OV/1, Gain2/1
  Gain4/1 -> Add4/1

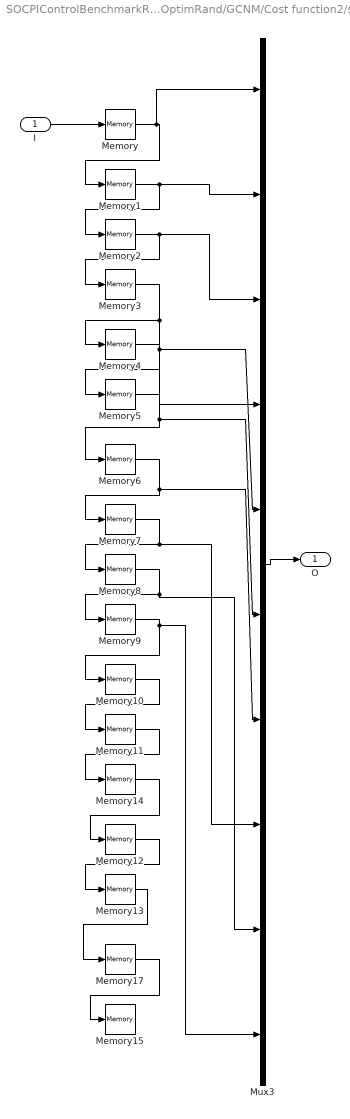
== system SOCPIControlBenchmarkRealDTOptimRand/GCNM/Cost function2/swY ==
  I : Inport
  Memory{,1..15,17} (17 alike) : Memory
  Mux3 : Mux  Inputs=10
  O : Outport
  wires:
  Memory11/1 -> Memory14/1
  Memory14/1 -> Memory12/1
  Memory12/1 -> Memory13/1
  Memory13/1 -> Memory17/1
  Memory5/1 -> Memory6/1, Mux3/6
  Memory4/1 -> Memory5/1, Mux3/5
  Mux3/1 -> O/1
  Memory9/1 -> Memory10/1, Mux3/10
  Memory3/1 -> Memory4/1, Mux3/4
  Memory6/1 -> Memory7/1, Mux3/7
  Memory1/1 -> Memory2/1, Mux3/2
  Memory10/1 -> Memory11/1
  Memory2/1 -> Memory3/1, Mux3/3
  I/1 -> Memory/1
  Memory8/1 -> Memory9/1, Mux3/9
  Memory/1 -> Memory1/1, Mux3/1
  Memory7/1 -> Memory8/1, Mux3/8
  Memory17/1 -> Memory15/1
